simulink library "biped_lib"  (R2020b)
settings: Solver=VariableStepAuto  StartTime=0.0  StopTime=10.0  RelTol=1e-3
values from neighbouring files (symbols this model uses):
  Ts = 1/fs    (= 0.001)    [bipedal.m]
undefined symbols (not defined in the file or in its folder): foot, Kd, Kf, Ki, Kp, sim_floor, use_integrator, X, Y, Z
libraries: nesl_utility x39, sm_lib x25, $bdroot x2, Contact_Forces_Lib x1
(part 2 of 2)

== system biped_lib/GasDamper/Translational joint ==
  No force : Subsystem  VariantControl=simulate_gas_sd == 0
  Spring-damper force : Subsystem  VariantControl=simulate_gas_sd == 1
  UpperPart : PMIOPort  Side=Left
  LowerPart : PMIOPort  Port=2  Side=Right

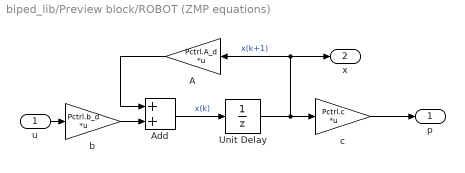
== system biped_lib/Preview block/ROBOT (ZMP equations) ==
  u : Inport
  A : Gain  Gain=Pctrl.A_d  Multiplication=Matrix(K*u)
  Add : Sum
  Unit Delay : UnitDelay  InitialCondition=[0,0,0]  SampleTime=Pctrl.Ts  HasFrameUpgradeWarning=on
  b : Gain  Gain=Pctrl.b_d  Multiplication=Matrix(K*u)
  c : Gain  Gain=Pctrl.c  Multiplication=Matrix(K*u)
  p : Outport
  x : Outport  Port=2
  wires:
  b/1 -> Add/2
  Add/1 -> Unit Delay/1  "x(k)"
  A/1 -> Add/1
  Unit Delay/1 -> c/1, A/1, x/1  "x(k+1)"
  u/1 -> b/1
  c/1 -> p/1

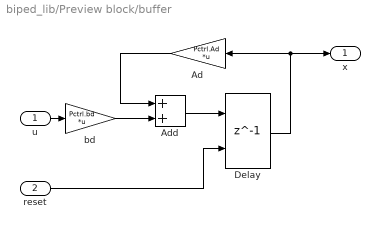
== system biped_lib/Preview block/buffer ==
  u : Inport
  reset : Inport  Port=2
  Ad : Gain  Gain=Pctrl.Ad  Multiplication=Matrix(K*u)
  Add : Sum
  Delay : Delay  DelayLength=1  InitialCondition=zeros(Pctrl.N_L,1)  ExternalReset=Rising  SampleTime=Pctrl.Ts
      settings: InputPortMap=u0,r5
  bd : Gain  Gain=Pctrl.bd  Multiplication=Matrix(K*u)
  x : Outport
  wires:
  u/1 -> bd/1
  Delay/1 -> x/1, Ad/1
  Ad/1 -> Add/1
  Add/1 -> Delay/1
  bd/1 -> Add/2
  reset/1 -> Delay/2

== system biped_lib/FootContact/Remapping of normal forces and ZMP computation/Bus to Mux ==
  Full contact data : Inport
  Mux : Mux
  Normal force selector : BusSelector  OutputSignals=fz1.Normal Force,fz2.Normal Force,fz3.Normal Force,fz4.Normal Force
  Normal forces only : Outport
  wires:
  Normal force selector/1 -> Mux/1  "<Normal Force>"
  Normal force selector/4 -> Mux/4  "<Normal Force>"
  Full contact data/1 -> Normal force selector/1
  Mux/1 -> Normal forces only/1
  Normal force selector/2 -> Mux/2  "<Normal Force>"
  Normal force selector/3 -> Mux/3  "<Normal Force>"

== system biped_lib/GasDamper/Translational joint/No force ==
  TranslationalJoint : sm_lib/Joints/Prismatic Joint  JointMode=Normal  SenseConstraintForce=off  SenseConstraintForceX=off  SenseConstraintForceY=off  SenseConstraintForceZ=off  SenseConstraintTorque=off  SenseConstraintTorqueX=off  SenseConstraintTorqueY=off  SenseConstraintTorqueZ=off  SenseTotalForce=off  SenseTotalForceX=off  SenseTotalForceY=off  SenseTotalForceZ=off  SenseTotalTorque=off  SenseTotalTorqueX=off  SenseTotalTorqueY=off  SenseTotalTorqueZ=off  CompositeWrenchDir=FollowerOnBase  CompositeWrenchFrame=BaseFrame  EquilibriumPosition=0  EquilibriumPositionUnits=m  SpringStiffness=0  SpringStiffnessUnits=N/m  DampingCoefficient=0  DampingCoefficientUnits=N/(m/s)  TorqueActuationMode=NoTorque  MotionActuationMode=ComputedMotion  SensePosition=off  SenseVelocity=off  SenseAcceleration=off  SenseTorqueForce=off  SenseLowerLimitTorqueForce=off  SenseUpperLimitTorqueForce=off  LowerLimitSpecify=on  LowerLimitBound=mech.tra.lim.min  LowerLimitBoundUnits=m  LowerLimitStiffness=1e6  LowerLimitStiffnessUnits=N/m  LowerLimitDamping=1e3  LowerLimitDampingUnits=N/(m/s)  LowerLimitTransitionRegionWidth=1e-4  LowerLimitTransitionRegionWidthUnits=m  UpperLimitSpecify=on  UpperLimitBound=mech.tra.lim.max  UpperLimitBoundUnits=m  UpperLimitStiffness=1e6  UpperLimitStiffnessUnits=N/m  UpperLimitDamping=1e3  UpperLimitDampingUnits=N/(m/s)  UpperLimitTransitionRegionWidth=1e-4  UpperLimitTransitionRegionWidthUnits=m  PositionTargetSpecify=off  PositionTargetPriority=High  PositionTargetValue=0  PositionTargetValueUnits=m  VelocityTargetSpecify=off  VelocityTargetPriority=High  VelocityTargetValue=0  VelocityTargetValueUnits=m/s
  UpperPart : PMIOPort  Side=Left
  LowerPart : PMIOPort  Port=2  Side=Right
  connections:
  TranslationalJoint/LConn1 -- UpperPart/RConn1
  TranslationalJoint/RConn1 -- LowerPart/RConn1

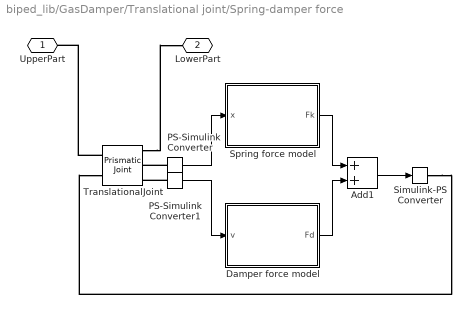
== system biped_lib/GasDamper/Translational joint/Spring-damper force ==
  Add1 : Sum
  Damper force model : Subsystem
  PS-Simulink Converter : nesl_utility/PS-Simulink Converter  PhysicalDomain=network_engine_domain  SubClassName=ps_output  LeftPortType=input  RightPortType=output  PseudoPeriodic=off  Frequencies=[]  Unit=inherit  AffineConversion=off
      settings: SourceProductName=Utilities
  PS-Simulink Converter1 : nesl_utility/PS-Simulink Converter  PhysicalDomain=network_engine_domain  SubClassName=ps_output  LeftPortType=input  RightPortType=output  PseudoPeriodic=off  Frequencies=[]  Unit=inherit  AffineConversion=off
      settings: SourceProductName=Utilities
  Simulink-PS Converter : nesl_utility/Simulink-PS Converter  PhysicalDomain=network_engine_domain  SubClassName=ps_input  LeftPortType=input  RightPortType=output  PseudoPeriodic=off  Frequencies=[]  NoiseDistribution=none  NoiseParameters=[]  Unit=1  AffineConversion=off  FilteringAndDerivatives=provide  SimscapeFilterOrder=1  InputFilterTimeConstant=0.001  UdotUserProvided=0
      settings: SourceProductName=Utilities
  Spring force model : Subsystem
  TranslationalJoint : sm_lib/Joints/Prismatic Joint  JointMode=Normal  SenseConstraintForce=off  SenseConstraintForceX=off  SenseConstraintForceY=off  SenseConstraintForceZ=off  SenseConstraintTorque=off  SenseConstraintTorqueX=off  SenseConstraintTorqueY=off  SenseConstraintTorqueZ=off  SenseTotalForce=off  SenseTotalForceX=off  SenseTotalForceY=off  SenseTotalForceZ=off  SenseTotalTorque=off  SenseTotalTorqueX=off  SenseTotalTorqueY=off  SenseTotalTorqueZ=off  CompositeWrenchDir=FollowerOnBase  CompositeWrenchFrame=BaseFrame  EquilibriumPosition=0  EquilibriumPositionUnits=m  SpringStiffness=0  SpringStiffnessUnits=N/m  DampingCoefficient=0  DampingCoefficientUnits=N/(m/s)  TorqueActuationMode=InputTorque  MotionActuationMode=ComputedMotion  SensePosition=on  SenseVelocity=on  SenseAcceleration=off  SenseTorqueForce=off  SenseLowerLimitTorqueForce=off  SenseUpperLimitTorqueForce=off  LowerLimitSpecify=on  LowerLimitBound=mech.tra.lim.min  LowerLimitBoundUnits=m  LowerLimitStiffness=1e6  LowerLimitStiffnessUnits=N/m  LowerLimitDamping=1e3  LowerLimitDampingUnits=N/(m/s)  LowerLimitTransitionRegionWidth=1e-4  LowerLimitTransitionRegionWidthUnits=m  UpperLimitSpecify=on  UpperLimitBound=mech.tra.lim.max  UpperLimitBoundUnits=m  UpperLimitStiffness=1e6  UpperLimitStiffnessUnits=N/m  UpperLimitDamping=1e3  UpperLimitDampingUnits=N/(m/s)  UpperLimitTransitionRegionWidth=1e-4  UpperLimitTransitionRegionWidthUnits=m  PositionTargetSpecify=off  PositionTargetPriority=High  PositionTargetValue=0  PositionTargetValueUnits=m  VelocityTargetSpecify=off  VelocityTargetPriority=High  VelocityTargetValue=0  VelocityTargetValueUnits=m/s
  UpperPart : PMIOPort  Side=Left
  LowerPart : PMIOPort  Port=2  Side=Right
  wires:
  Add1/1 -> Simulink-PS Converter/1
  PS-Simulink Converter/1 -> Spring force model/1(x)
  Spring force model/1(Fk) -> Add1/1
  PS-Simulink Converter1/1 -> Damper force model/1(v)
  Damper force model/1(Fd) -> Add1/2
  connections:
  TranslationalJoint/LConn1 -- UpperPart/RConn1
  TranslationalJoint/RConn1 -- LowerPart/RConn1
  PS-Simulink Converter/LConn1 -- TranslationalJoint/RConn2
  PS-Simulink Converter1/LConn1 -- TranslationalJoint/RConn3
  Simulink-PS Converter/RConn1 -- TranslationalJoint/LConn2

== system biped_lib/GasDamper/Translational joint/Spring-damper force/Damper force model ==
  v : Inport
  Gain2 : Gain  Gain=-mech.tra.mod.D
  Fd : Outport
  wires:
  v/1 -> Gain2/1
  Gain2/1 -> Fd/1  "Fd"

== system biped_lib/GasDamper/Translational joint/Spring-damper force/Spring force model ==
  x : Inport
  Add : Sum  Inputs=-+
  Constant : Constant
  Gain : Gain  Gain=mech.tra.mod.F0
  Gain1 : Gain  Gain=1/2*mech.tra.mod.L0
  Fk : Outport
  wires:
  Add/1 -> Gain/1
  Gain1/1 -> Add/1
  Gain/1 -> Fk/1  "Fk"
  Constant/1 -> Add/2
  x/1 -> Gain1/1

== matlab function biped_lib/FootContact/Remapping of normal forces and ZMP computation/Recalculate feet force ==
  data: Fn input; AinvX input; AinvY input; Apseud input; Pe input; Fm output; Pm input; zmp output; state output; Rfoot2world input; tfoot2world input
function [Fm,zmp,state] = fcn(Fn,AinvX,AinvY,Apseud,Pe,Pm, Rfoot2world, tfoot2world)
    thr = 0; %threshold in newtons
    % get measured forces (F1 - up left, F2 - up right, F3 - down right, F4
    % - down left), global ZMP of the foot and the state of the contact
    % (1=no contact, 2=point contact, 3=edge contact, 4=full contact)
    [Fm,zmp,zmploc,state] = force_remapping(Fn,AinvX,AinvY,Apseud,Pe,Pm, Rfoot2world, tfoot2world,thr,'o');
end

== matlab function biped_lib/HEBI actuator/Acceleration measurement model ==
  data: R input; a_glo input; a_loc output; w_glo input; w_loc output
function [a_loc,w_loc] = fcn(R,a_glo,w_glo)
    g_glo = [0, 0, -9.81]'; %global gravity vector
    R_w_imu = reshape(R,3,3); %from imu frame to world
    R_imu_w = R_w_imu'; %from world to imu
    a_loc = R_imu_w*(a_glo+g_glo); %transform to the local frame
    w_loc = R_imu_w*w_glo; %transform to the local frame

== matlab function biped_lib/Link dynamic reference/skew symmetric matrix ==
  data: omega input; omega_skew output
function omega_skew = fcn(omega)
omega_skew = [
    0,omega(3),-omega(2);
    -omega(3),0,omega(1);
    omega(2),-omega(1),0
];
